simulink model "PMSM_MTPA"  (R2023b)
settings: Solver=VariableStepAuto  StartTime=0.0  StopTime=5  RelTol=1e-3
PostLoadFcn:
  | modelDir = fileparts(get_param(bdroot,'FileName')); tableFile = fullfile(modelDir,'mtpa_lookup_tables.mat'); if exist(tableFile,'file')   s = load(tableFile,'Te_table','id_table','iq_table');   assignin('base','Te_table',s.Te_table);   assignin('base','id_table',s.id_table);   assignin('base','iq_table',s.iq_table); end
InitFcn:
  | modelDir = fileparts(get_param(bdroot,'FileName')); tableFile = fullfile(modelDir,'mtpa_lookup_tables.mat'); if exist(tableFile,'file')   s = load(tableFile,'Te_table','id_table','iq_table');   assignin('base','Te_table',s.Te_table);   assignin('base','id_table',s.id_table);   assignin('base','iq_table',s.iq_table); end
libraries: powerlib_extras x3, spsCurrentMeasurementLib x1, spsDCVoltageSourceLib x1, spsGroundLib x1, spsUniversalBridgeLib x1, spsPermanentMagnetSynchronousMachineLib x1, spsSVPWMGenerator2LevelLib x1, SignalEditorBlockLib x1, spsabctodq0Lib x1, spsdq0toAlphaBetaZeroLib x1, spspowerguiLib x1
settings Model: Creator=asus  LastModifiedBy=asus

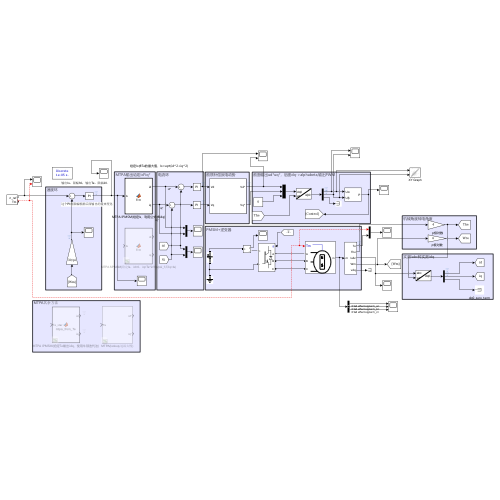
[thumbnail: Simulink's stored preview of the top-level diagram]
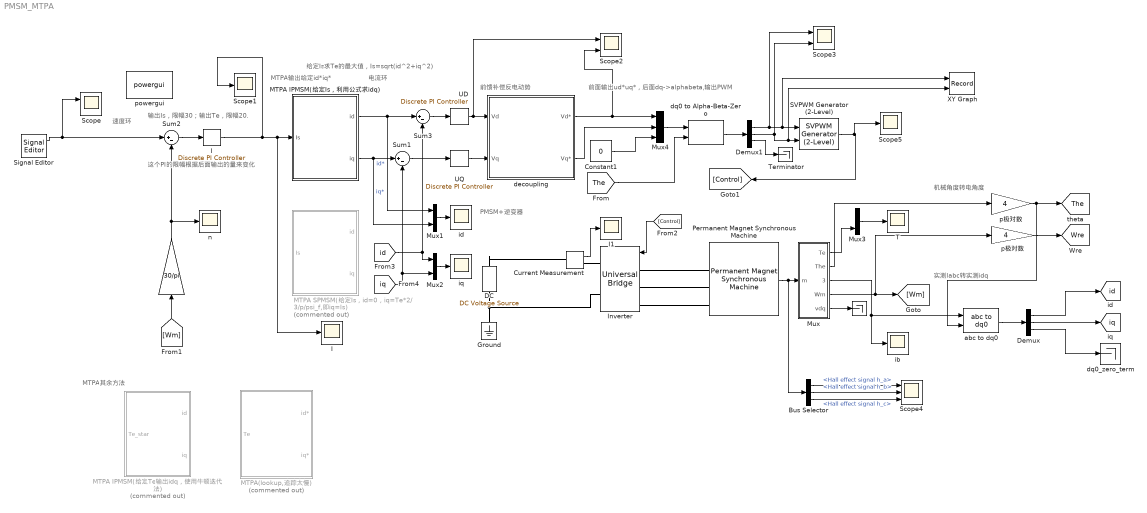
== system PMSM_MTPA ==
  note: MTPA其余方法
  note: 输出Is，限幅30；输出Te，限幅20.
  note: 这个PI的限幅根据后面输出的量来变化
  note: 前面输出ud*uq*，后面dq->alphabeta,输出PWM
  note: 实测Iabc转实测idq
  note: 电流环
  note: 机械角度转电角度
  note: PMSM+逆变器
  note: MTPA输出给定id*iq*
  note: 前馈补偿反电动势
  note: 给定Is求Te的最大值，Is=sqrt(id^2+iq^2)
  note: 速度环
  "  " : Gain  Gain=30/pi
  "         " : Terminator
  "   p极对数" : Gain  Gain=4
  "   p极对数   " : Gain  Gain=4
  Bus Selector : BusSelector  OutputSignals=Hall effect signal h_a,Hall effect signal h_b,Hall effect signal h_c
  Constant1 : Constant  Value=0
  Current Measurement : spsCurrentMeasurementLib/Current Measurement  PhasorSimulation=off  OutputType=Complex  PSBequivalent=0
  DC : spsDCVoltageSourceLib/DC Voltage Source  Amplitude=200  Measurements=None
  Demux : Demux  Outputs=3
  Demux1 : Demux  Outputs=3
  Ground : spsGroundLib/Ground  LConnTagsString=a
  I : Scope
  "I  " : powerlib_extras/Discrete  Control Blocks/Discrete PI Controller  Kp=6  Ki=15  Par_Limits=[30 0]  Init=0  Ts=1e-5
  I1 : Scope
  Inverter : spsUniversalBridgeLib/Universal Bridge  Arms=3  SnubberResistance=1e5  SnubberCapacitance=inf  Device=IGBT / Diodes  Ron=1e-3  Lon=0  ForwardVoltages="[  0  0  ]"  ForwardVoltage=0  GTOparameters=[ 10e-6 , 20e-6 ]  IGBTparameters=[ 1e-6 , 2e-6 ]  Measurements=None  Measurements_2=None  converterType=Rectifier
  MTPA IPMSM(给定Is，利用公式求idq) : MATLAB Function  TreatAsAtomicUnit=on
  MTPA IPMSM(给定Te输出idq，使用牛顿迭代法) : MATLAB Function  Commented=on  TreatAsAtomicUnit=on
  MTPA SPMSM(给定Is，id=0，iq=Te*2/3/p/psi_f,即iq=Is) : MATLAB Function  Commented=on  TreatAsAtomicUnit=on
  MTPA(lookup,追踪太慢) : Subsystem  Commented=on
  Mux : Subsystem
  Mux1 : Mux  Inputs=2
  Mux2 : Mux  Inputs=2
  Mux3 : Mux  Inputs=2
  Mux4 : Mux  Inputs=3
  Permanent Magnet Synchronous Machine : spsPermanentMagnetSynchronousMachineLib/Permanent Magnet Synchronous Machine  NbPhases=3  FluxDistribution=Sinusoidal  RotorType=Salient-pole  MechanicalLoad=Torque Tm  PresetModel=No  ShowDetailedParameters=on  MeasurementBus=off  Resistance=0.025  Inductance=8.5e-3  dqInductances=[0.2e-3,0.47e-3]  La=0.000835  MachineConstant=Flux linkage established by magnets (V.s)  Flux=0.062  VoltageCst=44.9822  TorqueCst=0.372  Flat=120  Mechanical=[0.01 0 4 0]  PolePairs=3  InitialConditions=[0,0, 0,0]  InitialConditions5ph=[0 0 0 0 0 0]  RefAngle=Aligned with phase A axis (original Park)  IterativeDiscreteModel=Trapezoidal non iterative  TsBlock=1e-5  TsPowergui=0
  SVPWM Generator (2-Level) : spsSVPWMGenerator2LevelLib/SVPWM Generator (2-Level)  InputType=alpha-beta components  SwitchingPattern=Pattern #1  Fc=10000  ParUref=[0.8 -30 50]  Ts=1e-5
  Scope : Scope  NumInputPorts=2
  Scope1 : Scope
  Scope2 : Scope  NumInputPorts=2
  Scope3 : Scope  NumInputPorts=2
  Scope4 : Scope  NumInputPorts=3
  Scope5 : Scope
  Signal Editor : SignalEditorBlockLib/Signal Editor  FileName=C:\Users\asus\Desktop\PMSM MTPA\scenario.mat  ActiveScenario=Scenario4  ActiveSignal=n_ref  IsBus=off  OutputBusObjectStr=Bus: BusObject  SampleTime=0  ZeroCross=off  OutputAfterFinalValue=Setting to zero  Unit=inherit  PreserveSignalName=on  ApplySigPropsToAllScenarios=on  ApplySigPropsToAllSignals=off
  Sum1 : Sum  Inputs=|+-
  Sum2 : Sum  Inputs=|+-
  Sum3 : Sum  Inputs=|+-
  T : Scope
  Terminator : Terminator
  UD : powerlib_extras/Discrete  Control Blocks/Discrete PI Controller  Kp=40  Ki=4333  Par_Limits=[200/sqrt(3) -200/sqrt(3)]  Init=0  Ts=1e-5
  UQ : powerlib_extras/Discrete  Control Blocks/Discrete PI Controller  Kp=100  Ki=4333  Par_Limits=[200/sqrt(3) -200/sqrt(3)]  Init=0  Ts=1e-5
  XY Graph : Record  FileSettingsInternal="{\"entries\":[{\"content\":{\"excelSettings\":{\"content\":{},\"type\":\"Streamout.ExcelSettings\"}},\"type\":\"Streamout.FileSettingStorage\",\"uuid\":\"\"}],\"packageUris\":[\"http:\\/\\/schema.mathworks.com\\/mf0\\/streamout_blocks\\/R2020a\"],\"version\":\"1.0\"}"  Layout=[1 1]  SignalsInternal="{\"entries\":[{\"content\":{\"signals\":[{\"content\":{\"blockPath\":[],\"dimensions\":[1],\"domain\":\"\",\"lineColor\":\"#a2142f\",\"plots\":[1],\"port\":1,\"signalID\":8,\"signalName\":\"Demux1:1\"},\"type\":\"RecordBlkView.Signal\",\"uuid\":\"\"},{\"content\":{\"blockPath\":[],\"dimensions\":[1],\"domain\":\"\",\"lineColor\":\"#139fff\",\"plots\":[1],\"port\":2,\"signalID\":11,\"signalName\":\"Demux1:2\"},\"type\":\"RecordBlkView.Signal\",\"uuid\":\"\"}]},\"type\":\"RecordBlkView.InputSignals\",\"uuid\":\"\"}],\"packageUris\":[\"http:\\/\\/schema.mathworks.com\\/mf0\\/streamout_blocks\\/R2020a\"],\"version\":\"1.0\"}"  VisualizationBindings="{\"xyplotplugin\":{\"info\":[{\"series\":[{\"bindingParametersList\":[{\"parameter\":\"X-Axis\",\"signalID\":8,\"signalName\":\"Demux1:1\"},{\"parameter\":\"Y-Axis\",\"signalID\":11,\"signalName\":\"Demux1:2\"}],\"seriesID\":25525}],\"subplotID\":1}]}}"  CompatibilityTag=XY
  abc to dq0 : spsabctodq0Lib/abc to dq0  Alignment=Aligned with phase A axis
  decoupling : Subsystem
  dq0 to Alpha-Beta-Zero : spsdq0toAlphaBetaZeroLib/dq0 to Alpha-Beta-Zero  Alignment=Aligned with phase A axis
  dq0_zero_term : Terminator
  ib : Scope
  "id " : Scope
  "iq " : Scope
  n : Scope
  powergui : spspowerguiLib/powergui  Priority=1  SimulationMode=Discrete  SampleTime=1e-5  frequency=60  Iterations=50  frequencyindice=0  Pbase=100e6  ErrMax=1e-4  UnitsV=kV  UnitsW=MW  buscounter=0  FunctionMessages=off  echomessages=off  EnableUseOfTLC=off  CurrentSourceSwitches=off  DisableSnubberDevices=off  DisableRonSwitches=off  DisableVfSwitches=off  DisplayEquations=off  AutomaticDiscreteSolvers=off  SolverType=Tustin  Interpol=off  ExternalGateDelay=off  methode=off  Ts=0  x0status=blocks  SPID=off  SwTol=0  HookPort=off  NonlinearTolerance=1e-4  nMaxIteration=100  ContinueOnMaxIteration=off  RestoreLinks=warning  ResistiveCurrentMeasurement=off  Frange=[0:2:500]  Ylog=off  Xlog=on  ShowGrid=off  save=off  variable=ZData  structure=n1  ZoomFFT=off  StartTime=0.0  cycles=1  DisplayStyle=1  fundamental=60  FreqAxis=off  MaxFrequency=1000  frequencyindicesteady=1  RmsSteady=1  display=off
  tag scope: The=global, Wre=global, id=global, iq=global
  wires:
  abc to dq0/1 -> Demux/1
  dq0 to Alpha-Beta-Zero/1 -> Demux1/1
  Mux/3(Iabc) -> ib/1, abc to dq0/1
  [The] -> dq0 to Alpha-Beta-Zero/2
  Signal Editor/1 -> Scope/1, Sum2/1
  [iq] -> Mux2/2, Sum1/2
  Demux/2 -> [iq]
  SVPWM Generator (2-Level)/1 -> Scope5/1, [Control]
  Mux2/1 -> "iq "/1
  Mux1/1 -> "id "/1
  Permanent Magnet Synchronous Machine/1 -> Bus Selector/1, Mux/1(m)
  Demux/1 -> [id]
  [Control] -> Inverter/1
  Mux/1(Te) -> Mux3/2
  Mux/5(vdq) -> "         "/1
  MTPA IPMSM(给定Is，利用公式求idq)/1(id) -> Mux1/1, Sum3/1  "id*"
  Current Measurement/1 -> I1/1
  Constant1/1 -> Mux4/3
  [Wm] -> "  "/1
  Mux4/1 -> dq0 to Alpha-Beta-Zero/1
  Demux1/3 -> Terminator/1
  Demux1/1 -> Scope3/1, XY Graph/1, SVPWM Generator (2-Level)/1
  MTPA IPMSM(给定Is，利用公式求idq)/2(iq) -> Mux1/2, Sum1/1  "iq*"
  Demux1/2 -> Scope3/2, XY Graph/2, SVPWM Generator (2-Level)/2
  decoupling/1(Vd*) -> Scope2/2, Mux4/1
  decoupling/2(Vq*) -> Mux4/2
  [id] -> Sum3/2, Mux2/1
  UD/1 -> Scope2/1, decoupling/1(Vd)
  Sum2/1 -> "I  "/1
  UQ/1 -> decoupling/2(Vq)
  "I  "/1 -> Scope1/1, I/1, MTPA IPMSM(给定Is，利用公式求idq)/1(Is)
  Mux/4(Wm) -> [Wm], "   p极对数   "/1
  "   p极对数   "/1 -> [Wre]
  Sum3/1 -> UD/1
  Mux3/1 -> T/1
  "   p极对数"/1 -> [The], abc to dq0/2
  Sum1/1 -> UQ/1
  "  "/1 -> n/1, Sum2/2
  Mux/2(The) -> "   p极对数"/1
  Demux/3 -> dq0_zero_term/1
  ? -> Scope/2, Mux3/1, Permanent Magnet Synchronous Machine/1
  Bus Selector/1 -> Scope4/1  "<Hall effect signal h_a>"
  Bus Selector/2 -> Scope4/2  "<Hall effect signal h_b>"
  Bus Selector/3 -> Scope4/3  "<Hall effect signal h_c>"
  connections:
  Inverter/RConn2 -- DC/LConn1 -- Ground/LConn1
  DC/RConn1 -- Current Measurement/LConn1
  Inverter/LConn1 -- Permanent Magnet Synchronous Machine/LConn1
  Inverter/LConn3 -- Permanent Magnet Synchronous Machine/LConn3
  Inverter/LConn2 -- Permanent Magnet Synchronous Machine/LConn2
  Current Measurement/RConn1 -- Inverter/RConn1

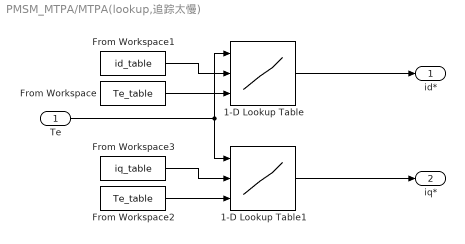
== system PMSM_MTPA/MTPA(lookup,追踪太慢) ==
  Te : Inport
  1-D Lookup Table : Lookup_n-D  NumberOfTableDimensions=1  BreakpointsForDimension1Source=Input port  BreakpointsForDimension1=[-5:5]  TableSource=Input port  Table=tanh([-5:5])  InternalRulePriority=Speed  RndMeth=Simplest
      settings: InputPortMap=u0,p221,p5
  1-D Lookup Table1 : Lookup_n-D  NumberOfTableDimensions=1  BreakpointsForDimension1Source=Input port  BreakpointsForDimension1=[-5:5]  TableSource=Input port  Table=tanh([-5:5])  InternalRulePriority=Speed  RndMeth=Simplest
      settings: InputPortMap=u0,p221,p5
  From Workspace : FromWorkspace  VariableName=Te_table
  From Workspace1 : FromWorkspace  VariableName=id_table
  From Workspace2 : FromWorkspace  VariableName=Te_table
  From Workspace3 : FromWorkspace  VariableName=iq_table
  id* : Outport
  iq* : Outport  Port=2
  wires:
  1-D Lookup Table/1 -> id*/1
  From Workspace2/1 -> 1-D Lookup Table1/3
  From Workspace/1 -> 1-D Lookup Table/3
  1-D Lookup Table1/1 -> iq*/1
  From Workspace1/1 -> 1-D Lookup Table/2
  From Workspace3/1 -> 1-D Lookup Table1/2
  Te/1 -> 1-D Lookup Table/1, 1-D Lookup Table1/1

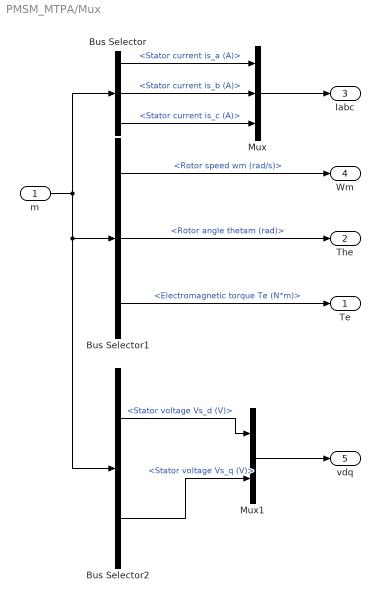
== system PMSM_MTPA/Mux ==
  m : Inport
  Bus Selector : BusSelector  OutputSignals=Stator current is_a (A),Stator current is_b (A),Stator current is_c (A)
  Bus Selector1 : BusSelector  OutputSignals=Rotor speed wm (rad/s),Rotor angle thetam (rad),Electromagnetic torque Te (N*m)
  Bus Selector2 : BusSelector  OutputSignals=Stator voltage Vs_d (V),Stator voltage Vs_q (V)
  Mux : Mux  Inputs=3
  Mux1 : Mux  Inputs=2
  Te : Outport
  The : Outport  Port=2
  Iabc : Outport  Port=3
  Wm : Outport  Port=4
  vdq : Outport  Port=5
  wires:
  Bus Selector1/1 -> Wm/1  "<Rotor speed wm (rad/s)>"
  Bus Selector1/2 -> The/1  "<Rotor angle thetam (rad)>"
  Bus Selector1/3 -> Te/1  "<Electromagnetic torque Te (N*m)>"
  m/1 -> Bus Selector/1, Bus Selector2/1, Bus Selector1/1
  Bus Selector/2 -> Mux/2  "<Stator current is_b (A)>"
  Bus Selector/3 -> Mux/3  "<Stator current is_c (A)>"
  Bus Selector/1 -> Mux/1  "<Stator current is_a (A)>"
  Mux/1 -> Iabc/1
  Bus Selector2/1 -> Mux1/1  "<Stator voltage Vs_d (V)>"
  Bus Selector2/2 -> Mux1/2  "<Stator voltage Vs_q (V)>"
  Mux1/1 -> vdq/1

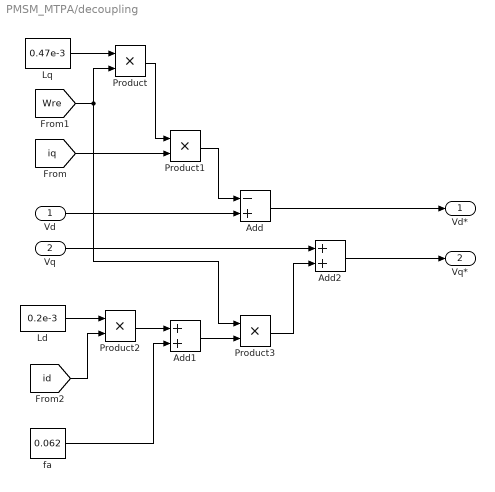
== system PMSM_MTPA/decoupling ==
  Vd : Inport
  Vq : Inport  Port=2
  Add : Sum  Inputs=-+
  Add1 : Sum
  Add2 : Sum
  Ld : Constant  Value=0.2e-3
  Lq : Constant  Value=0.47e-3
  Product{,1..3} (4 alike) : Product
  fa : Constant  Value=0.062
  Vd* : Outport
  Vq* : Outport  Port=2
  wires:
  Lq/1 -> Product/1
  [Wre] -> Product3/1, Product/2
  Product/1 -> Product1/1
  [iq] -> Product1/2
  Add/1 -> Vd*/1
  Product1/1 -> Add/1
  Vd/1 -> Add/2
  Ld/1 -> Product2/1
  [id] -> Product2/2
  Product2/1 -> Add1/1
  fa/1 -> Add1/2
  Add1/1 -> Product3/2
  Product3/1 -> Add2/2
  Vq/1 -> Add2/1
  Add2/1 -> Vq*/1

== matlab function PMSM_MTPA/MTPA IPMSM(给定Te输出idq，使用牛顿迭代法) ==
  data: Te_star input; id output; iq output
function [id, iq] = mtpa_from_Te(Te_star)
% 牛顿迭代法在线求解
Ld=0.2e-3;
Lq=0.47e-3;
psi_f=0.062;
p=4;
% 初值

iq = Te_star / (1.5 * p * psi_f);
id = 0;

for iter = 1:10
    % MTPA 条件
    id_new = psi_f/(2*(Lq-Ld)) - sqrt(psi_f^2/(4*(Lq-Ld)^2) + iq^2);
    % 转矩约束反解
    iq_new = Te_star / (1.5 * p * (psi_f + (Ld - Lq) * id));
    % 收敛判断
    if abs(id_new - id) < 1e-6 && abs(iq_new - iq) < 1e-6
        break;
    end
    id = id_new;
    iq = iq_new;
end
end

== matlab function PMSM_MTPA/MTPA SPMSM(给定Is，id=0，iq=Te*2//3//p//psi_f,即iq=Is) ==
  data: Is input; id output; iq output
function [id,iq] = fcn(Is)
%#codegen
id=0;
iq=Is;

== matlab function PMSM_MTPA/MTPA IPMSM(给定Is，利用公式求idq) ==
  data: Is input; id output; iq output
function [id,iq] = fcn(Is)
%#codegen
Ld=0.2e-3;
Lq=0.47e-3;
posaif=0.062;
id=(posaif-sqrt(posaif^2+8*(Ld-Lq)^2*Is^2))/(4*(Lq-Ld));
iq=sqrt(Is^2-id^2);
